simulink model "mpc_simulink"  (R2024a)
settings: Solver=VariableStepAuto  StartTime=0.0  StopTime=10  RelTol=1e-3
libraries: mpclib x1
settings Model: Creator=Siddarth  LastModifiedBy=Siddarth

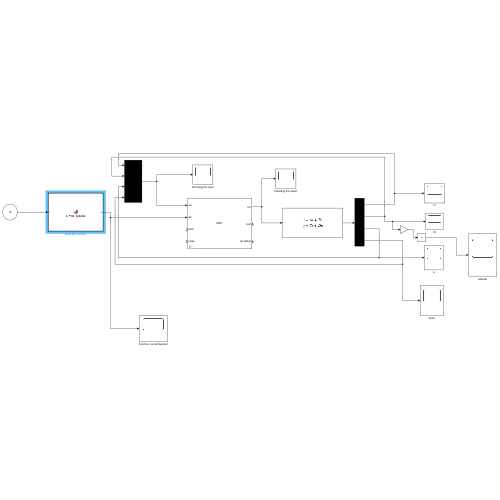
[thumbnail: Simulink's stored preview of the top-level diagram]
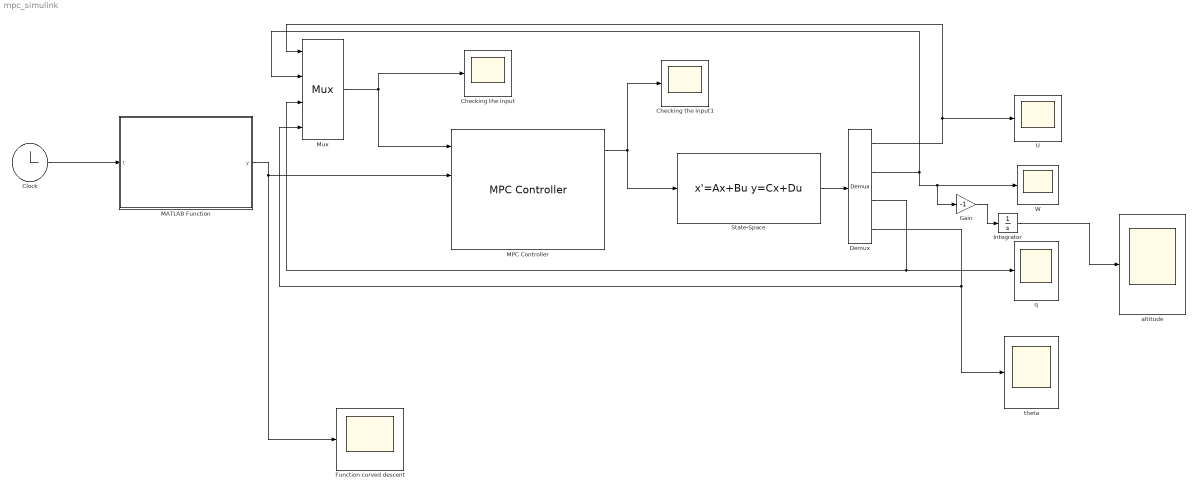
== system mpc_simulink ==
  Checking the input : Scope
  Checking the input1 : Scope
  Clock : Clock
  Demux : Demux
  Function curved descent : Scope
  Gain : Gain  Gain=-1
  Integrator : Integrator  InitialCondition=10000
  MATLAB Function : MATLAB Function  TreatAsAtomicUnit=on
  MPC Controller : mpclib/MPC Controller  SCDEnableBlockLinearizationSpecification=on  is_multiple=0  enable_value=0  return_u0=off  updateMPCinCallerWorkspace=on  md_inport=off  mv_inport=off  uref_inport=off  return_cost=on  return_mvseq=off  return_qpstatus=on  return_xseq=off  return_state=off  return_ovseq=off  state_inport=off  umin_inport=on  umax_inport=on  ymin_inport=off  ymax_inport=off  cc_inport=off  ywt_inport=off  uwt_inport=off  duwt_inport=off  rhoeps_inport=off  pm_inport=off  MaximumP=10  HorizonChoice=FixedHorizon  n_ts=0.01  n_p=50  n_mv=1  n_md=1  n_ud=0  n_mo=4  n_uo=0  BlockDataType=double  SampleTimeInherited=off  switch_inport=off
  Mux : Mux
  State-Space : StateSpace  A=|  B=[0; 9.748; 3.77; -0.034];  C=eye(4);  D=zeros(4,1);  InitialCondition=[20; 20; 20; 20]  ContinuousStateAttributes=|
      A=|
      | [-0.0089  -0.1474     0   -9.75;
      |      -0.0216  -0.3601   5.947  -0.151;
      |       0      -0.00015 -0.0224  0.0006;
      |       0       1         0       0];
      ContinuousStateAttributes=|
      | {'u','w','q','theta'
      | }
  U : Scope
  W : Scope
  altitude : Scope
  q : Scope
  theta : Scope
  wires:
  MPC Controller/1 -> State-Space/1, Checking the input1/1
  State-Space/1 -> Demux/1
  Demux/1 -> Mux/1, U/1
  Demux/3 -> Mux/3, q/1
  Demux/4 -> theta/1, Mux/4
  Demux/2 -> Mux/2, Gain/1, W/1
  Integrator/1 -> altitude/1
  Mux/1 -> Checking the input/1, MPC Controller/1
  Clock/1 -> MATLAB Function/1(t)
  MATLAB Function/1(y) -> Function curved descent/1, MPC Controller/2
  Gain/1 -> Integrator/1

== matlab function mpc_simulink/MATLAB Function ==
  data: t input; y output
function y = curved_descent(t)
    % y = [u_ref, w_ref, q_ref, theta_ref];

    w0 = -300;               % final vertical velocity
    theta0 = deg2rad(-45);   % final pitch angle
    tf = 80;

    w_ref = w0 * (1 - cos(pi * t / tf)) / 2;
    theta_ref = theta0 * (1 - cos(pi * t / tf)) / 2;

    y = [0, w_ref, 0, theta_ref];  % row vector output [1x4]
end
